simulink model "SWC_HALOUT_type"  (R2021b)
settings: Solver=FixedStepDiscrete  StartTime=0.0  StopTime=10.0  FixedStep=0.005  RelTol=1e-3
undefined symbols (not defined in the file): DIDLen_APPD, DIDLen_APPE, DIDLen_APPPedalZP, DIDLen_APSFunConfig, DIDLen_AutoLock, DIDLen_AutoWipHSpdEN, DIDLen_CALID, DIDLen_CDEODT, DIDLen_CLRDIST, DIDLen_DKCBLESta, DIDLen_DKCKey, DIDLen_DKCSta, DIDLen_DoorNFCAnchorSta, DIDLen_DRLDis, DIDLen_DynoMode, DIDLen_ECUNAME, DIDLen_FDDKCCoordXY, DIDLen_FMHTimer, DIDLen_LFLowPresThre, DIDLen_LFSensorID, DIDLen_LIDAAnchorSta, DIDLen_LRLowPresThre, DIDLen_LRSensorID, DIDLen_MILDIST, DIDLen_NUMPSATRIPSFLTMEMCLR, DIDLen_NVMPedalZP, DIDLen_OBDReq, DIDLen_ODOMETER, DIDLen_PKE, DIDLen_ProtocolId, DIDLen_PSA, DIDLen_QTYPSATRIPS, DIDLen_RFLowPresThre, DIDLen_RFSensorID, DIDLen_RRLowPresThre, DIDLen_RRSensorID, DIDLen_RUNTM, DIDLen_SensorMode, DIDLen_TestGroup, DIDLen_TireSize, DIDLen_TPMSLearnSta, DIDLen_TurnLampFLThreCurr, DIDLen_TurnLampFRThreCurr, DIDLen_TurnLampRLThreCurr, DIDLen_TurnLampRRThreCurr, DIDLen_UIDSta, DIDLen_USSConfig, DIDLen_UWBAnchorSta, DIDLen_VIN, DIDLen_VSS, DIDLen_WhlPres, DIDLen_WhlSensorBattSta, DIDLen_WhlTmp, DIDLen_WipRLSCmdCutFilter, DIDLen_WipRLSCmdHoldFilter, DIDLen_XWDMode, DIDNum_APPD, DIDNum_APPE, DIDNum_APPPedalZP, DIDNum_APSFunConfig ... (+504)
libraries: simulink x893, FVT_lib x320, hdlsllib x6, hcu_lib x5, halout x1
(part 3 of 11)

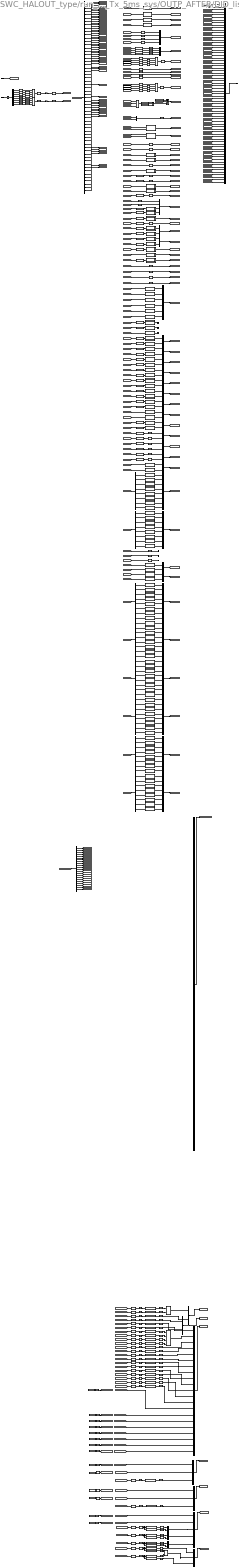
== system SWC_HALOUT_type/run_SWC_HALOUT_Tx_5ms_sys/OUTP_AFTER/DID_list ==
  BOUTP_outputs : Inport
  VHAL_NvmReadArray_raw : Inport  Port=2
  Bit Shift : hdlsllib/Logic and Bit Operations/Bit Shift  mode=Shift Left Logical  N=3
  Bit Shift1 : hdlsllib/Logic and Bit Operations/Bit Shift  mode=Shift Left Logical  N=2
  Bit Shift2 : hdlsllib/Logic and Bit Operations/Bit Shift  mode=Shift Left Logical  N=1
  Bit Shift3 : hdlsllib/Logic and Bit Operations/Bit Shift  mode=Shift Left Logical  N=3
  Bit Shift4 : hdlsllib/Logic and Bit Operations/Bit Shift  mode=Shift Left Logical  N=2
  Bit Shift5 : hdlsllib/Logic and Bit Operations/Bit Shift  mode=Shift Left Logical  N=1
  Bitwise OR : simulink/Logic and Bit Operations/Bitwise Operator  logicop=OR  UseBitMask=off  NumInputPorts=4  BitMask=bin2dec('11011001')  BitMaskRealWorld=Stored Integer
  Bitwise OR1 : simulink/Logic and Bit Operations/Bitwise Operator  logicop=OR  UseBitMask=off  NumInputPorts=4  BitMask=bin2dec('11011001')  BitMaskRealWorld=Stored Integer
  Bitwise OR13 : simulink/Logic and Bit Operations/Bitwise Operator  logicop=OR  UseBitMask=off  NumInputPorts=4  BitMask=bin2dec('00000000000000000000')  BitMaskRealWorld=Stored Integer
  Bitwise OR14 : simulink/Logic and Bit Operations/Bitwise Operator  logicop=OR  UseBitMask=off  NumInputPorts=4  BitMask=bin2dec('00000000000000000000')  BitMaskRealWorld=Stored Integer
  BitwiseAND : simulink/Logic and Bit Operations/Bitwise Operator  logicop=OR  UseBitMask=off  NumInputPorts=2  BitMask=bin2dec('11011001')  BitMaskRealWorld=Stored Integer
  BitwiseAND1 : simulink/Logic and Bit Operations/Bitwise Operator  logicop=OR  UseBitMask=off  NumInputPorts=4  BitMask=bin2dec('11011001')  BitMaskRealWorld=Stored Integer
  BitwiseAND2 : simulink/Logic and Bit Operations/Bitwise Operator  logicop=OR  UseBitMask=off  NumInputPorts=2  BitMask=bin2dec('11011001')  BitMaskRealWorld=Stored Integer
  Bus Creator : BusCreator  Inputs=71
  Bus Selector : BusSelector  OutputSignals=VOUTP_WriteChkLFID_raw,VOUTP_WriteChkRFID_raw,VOUTP_WriteChkLRID_raw,VOUTP_WriteChkRRID_raw,VOUTP_LFWheelPress_raw8,VOUTP_RFWheelPress_raw8,VOUTP_LRWheelPress_raw8,VOUTP_RRWheelPress_raw8,VOUTP_LFWheelTemp_C,VOUTP_RFWheelTemp_C,VOUTP_LRWheelTemp_C,VOUTP_RRWheelTemp_C,VOUTP_LFBatWarn_flg,VOUTP_RFBatWarn_flg,VOUTP_LRBatWarn_flg,VOUTP_RRBatWarn_flg,VOUTP_LFWheelPSW_raw8,VOUTP_LRWheelPSW_raw8,VOUTP_RFWheelPSW_raw8,VOUTP_RRWheelPSW_raw8,VOUTP_LFSensorMode_flg,VOUTP_RFSensorMode_flg,VOUTP_LRSensorMode_flg,VOUTP_RRSensorMode_flg,VOUTP_ALFin_flg,VOUTP_ChkStorge_flg,VOUTP_TPMSStorge_flg,VOUTP_unlearnSfali_flg,VOUTP_WritingCnt_enum,VOUTP_LProgress_enum,VOUTP_EAPS1MIN_pct,VOUTP_EAPS2MIN_pct,VOUTP_DrivetrainSelect_enum,VOUTP_VSS_kph,VOUTP_RUNTM_s,VOUTP_MILDIST_km,VOUTP_CLRDIST_km,VOUTP_APPD_pct,VOUTP_APPE_pct,VOUTP_ODOMETER_km,VOUTP_NUMPSATRIPSFLTMEMCLR_cnt,VOUTP_VinCode_cnt,VOUTP_CALID_cnt,VOUTP_ECUNAME_cnt,VOUTP_PROTOCOLID_enum,VOUTP_PSAR_sec,VOUTP_PSAL_sec,VOUTP_IPSAR_sec,VOUTP_IPSAL_sec,VOUTP_CPSAR_sec,VOUTP_CPSAL_sec,VOUTP_PKER_kphsqr,VOUTP_PKEL_kphsqr,VOUTP_CDEODTR_km,VOUTP_CDEODTL_km,VOUTP_QTYPSATRIPSR_cnt,VOUTP_QTYPSATRIPSL_cnt
  Constant : Constant  Value=ENUM_TPMSLearnStatus_LEARNFAIL
  Constant1 : Constant  Value=ENUM_TPMSLearnStatus_NOTLEARN
  Constant{3..16} (14 alike) : Constant  Value=zeros(10,1)
  Constant2 : Constant  Value=ENUM_TPMSLearnStatus_LEARNED
  Data Type Conversion{,1..58} (59 alike) : DataTypeConversion  OutDataTypeStr=uint8
  Data Type Conversion168 : DataTypeConversion  OutDataTypeStr=single
  Data Type Conversion{169..178} (10 alike) : DataTypeConversion  OutDataTypeStr=uint32
  Data Type Conversion179 : DataTypeConversion  OutDataTypeStr=single
  Demux{,1..8} (9 alike) : Demux  Outputs=8
  Logical Operator1 : Logic  Operator=OR  Inputs=3  AllPortsSameDT=off  OutDataTypeStr=boolean
  Multiply1 : Gain  Gain=1/10000
  Multiply2 : Gain  Gain=1/10000
  Mux : Mux
  Mux{1,4..5,7..19,22..23,37..38,58..60} (23 alike) : Mux  Inputs=2
  Mux2 : Mux
  Mux{20..21,24..29} (8 alike) : Mux  Inputs=8
  Mux3 : Mux
  Mux36 : Mux  Inputs=56
  Mux48 : Mux  Inputs=21
  Mux51 : Mux  Inputs=3
  Mux55 : Mux  Inputs=3
  Mux6 : Mux  Inputs=6
  Mux61 : Mux  Inputs=5
  Mux65 : Mux  Inputs=3
  Selector1 : Selector  InputPortWidth=1024  IndexOptions=Index vector (dialog)  Indices=[112:119]  OutputSizes=1
  Shift Arithmetic37 : ArithShift  BitShiftNumber=8  BitShiftDirection=Left
  Shift Arithmetic38 : ArithShift  BitShiftNumber=16  BitShiftDirection=Left
  Shift Arithmetic39 : ArithShift  BitShiftNumber=24  BitShiftDirection=Left
  Shift Arithmetic40 : ArithShift  BitShiftNumber=8  BitShiftDirection=Left
  Shift Arithmetic41 : ArithShift  BitShiftNumber=16  BitShiftDirection=Left
  Shift Arithmetic42 : ArithShift  BitShiftNumber=24  BitShiftDirection=Left
  SignalPack181 : FVT_lib/hal/SignalPack_shiftAfterMask  RightShiftCnt=0  BitMask=2^4-1  LeftShiftCnt=4
  SignalPack182 : FVT_lib/hal/SignalPack_shiftAfterMask  RightShiftCnt=0  BitMask=2^4-1  LeftShiftCnt=0
  SignalPack{183..186,192..201,302,323} (16 alike) : FVT_lib/hal/SignalPack_shiftAfterMask  RightShiftCnt=0  BitMask=2^8-1  LeftShiftCnt=0
  SignalPack187 : FVT_lib/hal/SignalPack_shiftAfterMask  RightShiftCnt=0  BitMask=2^2-1  LeftShiftCnt=6
  SignalPack188 : FVT_lib/hal/SignalPack_shiftAfterMask  RightShiftCnt=0  BitMask=2^2-1  LeftShiftCnt=4
  SignalPack189 : FVT_lib/hal/SignalPack_shiftAfterMask  RightShiftCnt=0  BitMask=2^2-1  LeftShiftCnt=2
  SignalPack190 : FVT_lib/hal/SignalPack_shiftAfterMask  RightShiftCnt=0  BitMask=2^2-1  LeftShiftCnt=0
  SignalPack191 : FVT_lib/hal/SignalPack_shiftAfterMask  RightShiftCnt=0  BitMask=2^2-1  LeftShiftCnt=0
  SignalPack344 : FVT_lib/hal/SignalPack_shiftAfterMask  RightShiftCnt=8  BitMask=65280  LeftShiftCnt=0
  SignalPack345 : FVT_lib/hal/SignalPack_shiftAfterMask  RightShiftCnt=0  BitMask=255  LeftShiftCnt=0
  SignalPack346 : FVT_lib/hal/SignalPack_shiftAfterMask  RightShiftCnt=8  BitMask=65280  LeftShiftCnt=0
  SignalPack347 : FVT_lib/hal/SignalPack_shiftAfterMask  RightShiftCnt=0  BitMask=255  LeftShiftCnt=0
  SignalPack348 : FVT_lib/hal/SignalPack_shiftAfterMask  RightShiftCnt=8  BitMask=65280  LeftShiftCnt=0
  SignalPack349 : FVT_lib/hal/SignalPack_shiftAfterMask  RightShiftCnt=0  BitMask=255  LeftShiftCnt=0
  SignalPack350 : FVT_lib/hal/SignalPack_shiftAfterMask  RightShiftCnt=1  BitMask=511  LeftShiftCnt=0
  SignalPack351 : FVT_lib/hal/SignalPack_shiftAfterMask  RightShiftCnt=0  BitMask=1  LeftShiftCnt=7
  SignalPack352 : FVT_lib/hal/SignalPack_shiftAfterMask  RightShiftCnt=2  BitMask=508  LeftShiftCnt=0
  SignalPack353 : FVT_lib/hal/SignalPack_shiftAfterMask  RightShiftCnt=0  BitMask=3  LeftShiftCnt=6
  Switch : Switch  Criteria=u2 ~= 0
  Switch1 : Switch  Criteria=u2 ~= 0
  Terminator_{1..6} (6 alike) : Terminator
  UnitConverter{237..278,389..390,413..414,438..439,441..442,444..445,447..448,450..451} (56 alike) : DataTypeConversion  OutDataTypeStr=uint8
  UnitConverter{437,440,443,446,449} (5 alike) : DataTypeConversion  OutDataTypeStr=uint16
  bus_selector : BusSelector  OutputSignals=VOUTP_KeyModeSta_enum,VOUTP_UWBDetArea_enum,VOUTP_BLERSSI_enum,VOUTP_UWBOnOff_flg,VOUTP_UWB1Invalid_flg,VOUTP_UWB2Invalid_flg,VOUTP_UWB3Invalid_flg,VOUTP_UWB4Invalid_flg,VOUTP_UWB0Invalid_flg,VOUTP_UWB1FPP_enum,VOUTP_UWB2FPP_enum,VOUTP_UWB3FPP_enum,VOUTP_UWB4FPP_enum,VOUTP_UWB0FPP_enum,VOUTP_UWB1Distance_enum,VOUTP_UWB2Distance_enum,VOUTP_UWB3Distance_enum,VOUTP_UWB4Distance_enum,VOUTP_UWB0Distance_enum,VOUTP_UIDBatVolt_enum,VOUTP_CoordinateX_enum,VOUTP_CoordinateY_enum
  convert_in{,5..13,17..21,25} (16 alike) : FVT_lib/hal/convert_in  gain=10  offset=0
  convert_in1 : FVT_lib/hal/convert_in  gain=1000  offset=2147483648
  convert_in{14..16,22..24} (6 alike) : FVT_lib/hal/convert_in  gain=1  offset=40
  convert_in2 : FVT_lib/hal/convert_in  gain=1000  offset=2147483648
  convert_in26 : FVT_lib/hal/convert_in  gain=1/0.015625  offset=0
  convert_in{27..30} (4 alike) : FVT_lib/hal/convert_in  gain=2.55  offset=0
  convert_in{3..4,31..32} (4 alike) : FVT_lib/hal/convert_in  gain=1000  offset=0
  convert_in33 : FVT_lib/hal/convert_in  gain=20  offset=0
  convert_in34 : FVT_lib/hal/convert_in  gain=20  offset=0
  convert_in35 : FVT_lib/hal/convert_in  gain=1000000  offset=2147483648
  convert_in36 : FVT_lib/hal/convert_in  gain=1000000  offset=2147483648
  convert_out{,1..3} (4 alike) : FVT_lib/hal/convert_out  gain=1  offset=-40
  convert_out100 : FVT_lib/hal/convert_out  gain=10  offset=-2550
  convert_out101 : FVT_lib/hal/convert_out  gain=10  offset=-2550
  convert_out{56..59,61..67,90,94} (13 alike) : FVT_lib/hal/convert_out  gain=1  offset=0
  convert_out{68..70,72..73} (5 alike) : FVT_lib/hal/convert_out  gain=1  offset=-127
  convert_out{74..78,97..99} (8 alike) : FVT_lib/hal/convert_out  gain=10  offset=0
  pct2raw1 : Subsystem
  pct2raw8 : Subsystem
  uint16Touint8Array1 : Subsystem
  uint16Touint8Array10 : Subsystem
  uint16Touint8Array11 : Subsystem
  uint16Touint8Array12 : Subsystem
  uint16Touint8Array13 : Subsystem
  uint16Touint8Array14 : Subsystem
  uint16Touint8Array15 : Subsystem
  uint16Touint8Array16 : Subsystem
  uint16Touint8Array17 : Subsystem
  uint16Touint8Array18 : Subsystem
  uint16Touint8Array19 : Subsystem
  uint16Touint8Array2 : Subsystem
  uint16Touint8Array20 : Subsystem
  uint16Touint8Array21 : Subsystem
  uint16Touint8Array22 : Subsystem
  uint16Touint8Array23 : Subsystem
  uint16Touint8Array24 : Subsystem
  uint16Touint8Array25 : Subsystem
  uint16Touint8Array26 : Subsystem
  uint16Touint8Array27 : Subsystem
  uint16Touint8Array28 : Subsystem
  uint16Touint8Array29 : Subsystem
  uint16Touint8Array3 : Subsystem
  uint16Touint8Array4 : Subsystem
  uint16Touint8Array5 : Subsystem
  uint16Touint8Array6 : Subsystem
  uint16Touint8Array7 : Subsystem
  uint16Touint8Array8 : Subsystem
  uint16Touint8Array9 : Subsystem
  uint32Touint8Array : Subsystem
  uint32Touint8Array1 : Subsystem
  uint32Touint8Array10 : Subsystem
  uint32Touint8Array11 : Subsystem
  uint32Touint8Array12 : Subsystem
  uint32Touint8Array13 : Subsystem
  uint32Touint8Array14 : Subsystem
  uint32Touint8Array15 : Subsystem
  uint32Touint8Array16 : Subsystem
  uint32Touint8Array17 : Subsystem
  uint32Touint8Array18 : Subsystem
  uint32Touint8Array19 : Subsystem
  uint32Touint8Array2 : Subsystem
  uint32Touint8Array20 : Subsystem
  uint32Touint8Array21 : Subsystem
  uint32Touint8Array22 : Subsystem
  uint32Touint8Array23 : Subsystem
  uint32Touint8Array24 : Subsystem
  uint32Touint8Array25 : Subsystem
  uint32Touint8Array26 : Subsystem
  uint32Touint8Array27 : Subsystem
  uint32Touint8Array28 : Subsystem
  uint32Touint8Array29 : Subsystem
  uint32Touint8Array3 : Subsystem
  uint32Touint8Array30 : Subsystem
  uint32Touint8Array31 : Subsystem
  uint32Touint8Array32 : Subsystem
  uint32Touint8Array33 : Subsystem
  uint32Touint8Array34 : Subsystem
  uint32Touint8Array35 : Subsystem
  uint32Touint8Array36 : Subsystem
  uint32Touint8Array37 : Subsystem
  uint32Touint8Array38 : Subsystem
  uint32Touint8Array39 : Subsystem
  uint32Touint8Array4 : Subsystem
  uint32Touint8Array40 : Subsystem
  uint32Touint8Array41 : Subsystem
  uint32Touint8Array42 : Subsystem
  uint32Touint8Array43 : Subsystem
  uint32Touint8Array44 : Subsystem
  uint32Touint8Array45 : Subsystem
  uint32Touint8Array46 : Subsystem
  uint32Touint8Array47 : Subsystem
  uint32Touint8Array48 : Subsystem
  uint32Touint8Array49 : Subsystem
  uint32Touint8Array5 : Subsystem
  uint32Touint8Array50 : Subsystem
  uint32Touint8Array51 : Subsystem
  uint32Touint8Array52 : Subsystem
  uint32Touint8Array53 : Subsystem
  uint32Touint8Array54 : Subsystem
  uint32Touint8Array55 : Subsystem
  uint32Touint8Array56 : Subsystem
  uint32Touint8Array57 : Subsystem
  uint32Touint8Array58 : Subsystem
  uint32Touint8Array59 : Subsystem
  uint32Touint8Array6 : Subsystem
  uint32Touint8Array60 : Subsystem
  uint32Touint8Array61 : Subsystem
  uint32Touint8Array62 : Subsystem
  uint32Touint8Array63 : Subsystem
  uint32Touint8Array64 : Subsystem
  uint32Touint8Array65 : Subsystem
  uint32Touint8Array66 : Subsystem
  uint32Touint8Array67 : Subsystem
  uint32Touint8Array68 : Subsystem
  uint32Touint8Array69 : Subsystem
  uint32Touint8Array7 : Subsystem
  uint32Touint8Array70 : Subsystem
  uint32Touint8Array71 : Subsystem
  uint32Touint8Array72 : Subsystem
  uint32Touint8Array73 : Subsystem
  uint32Touint8Array74 : Subsystem
  uint32Touint8Array75 : Subsystem
  uint32Touint8Array76 : Subsystem
  uint32Touint8Array77 : Subsystem
  uint32Touint8Array78 : Subsystem
  uint32Touint8Array79 : Subsystem
  uint32Touint8Array8 : Subsystem
  uint32Touint8Array80 : Subsystem
  uint32Touint8Array81 : Subsystem
  uint32Touint8Array82 : Subsystem
  uint32Touint8Array83 : Subsystem
  uint32Touint8Array84 : Subsystem
  uint32Touint8Array85 : Subsystem
  uint32Touint8Array86 : Subsystem
  uint32Touint8Array9 : Subsystem
  BOUTP_DIDSetData_outputs : Outport
  wires:
  Bus Selector/1 -> [VOUTP_WriteChkLFID_raw]  "<VOUTP_WriteChkLFID_raw>"
  Bus Selector/2 -> [VOUTP_WriteChkRFID_raw]  "<VOUTP_WriteChkRFID_raw>"
  Bus Selector/4 -> [VOUTP_WriteChkRRID_raw]  "<VOUTP_WriteChkRRID_raw>"
  Bus Selector/3 -> [VOUTP_WriteChkLRID_raw]  "<VOUTP_WriteChkLRID_raw>"
  Bus Selector/5 -> [VOUTP_LFWheelPress_raw8]  "<VOUTP_LFWheelPress_raw8>"
  Bus Selector/6 -> [VOUTP_RFWheelPress_raw8]  "<VOUTP_RFWheelPress_raw8>"
  Bus Selector/7 -> [VOUTP_LRWheelPress_raw8]  "<VOUTP_LRWheelPress_raw8>"
  Bus Selector/8 -> [VOUTP_RRWheelPress_raw8]  "<VOUTP_RRWheelPress_raw8>"
  Bus Selector/13 -> [VOUTP_LFBatWarn_flg]  "<VOUTP_LFBatWarn_flg>"
  Bus Selector/14 -> [VOUTP_RFBatWarn_flg]  "<VOUTP_RFBatWarn_flg>"
  Bus Selector/15 -> [VOUTP_LRBatWarn_flg]  "<VOUTP_LRBatWarn_flg>"
  Bus Selector/16 -> [VOUTP_RRBatWarn_flg]  "<VOUTP_RRBatWarn_flg>"
  Bus Selector/18 -> [VOUTP_LRWheelPSW_raw8]  "<VOUTP_LRWheelPSW_raw8>"
  Bus Selector/19 -> [VOUTP_RFWheelPSW_raw8]  "<VOUTP_RFWheelPSW_raw8>"
  Bus Selector/20 -> [VOUTP_RRWheelPSW_raw8]  "<VOUTP_RRWheelPSW_raw8>"
  Bus Selector/17 -> [VOUTP_LFWheelPSW_raw8]  "<VOUTP_LFWheelPSW_raw8>"
  Bus Selector/21 -> [VOUTP_LFSensorMode_flg]  "<VOUTP_LFSensorMode_flg>"
  Bus Selector/22 -> [VOUTP_RFSensorMode_flg]  "<VOUTP_RFSensorMode_flg>"
  Bus Selector/23 -> [VOUTP_LRSensorMode_flg]  "<VOUTP_LRSensorMode_flg>"
  Bus Selector/24 -> [VOUTP_RRSensorMode_flg]  "<VOUTP_RRSensorMode_flg>"
  Bus Selector/27 -> [VOUTP_TPMSStorge_flg]  "<VOUTP_TPMSStorge_flg>"
  Bus Selector/25 -> [VOUTP_ALFin_flg]  "<VOUTP_ALFin_flg>"
  Bus Selector/26 -> [VOUTP_ChkStorge_flg]  "<VOUTP_ChkStorge_flg>"
  Bus Selector/28 -> [VOUTP_unlearnSfali_flg]  "<VOUTP_unlearnSfali_flg>"
  Bus Selector/9 -> [VOUTP_LFWheelTemp_C]  "<VOUTP_LFWheelTemp_C>"
  Bus Selector/10 -> [VOUTP_RFWheelTemp_C]  "<VOUTP_RFWheelTemp_C>"
  Bus Selector/11 -> [VOUTP_LRWheelTemp_C]  "<VOUTP_LRWheelTemp_C>"
  Bus Selector/12 -> [VOUTP_RRWheelTemp_C]  "<VOUTP_RRWheelTemp_C>"
  Data Type Conversion8/1 -> Mux2/1
  Data Type Conversion9/1 -> Mux2/2
  Data Type Conversion10/1 -> Mux2/3
  Data Type Conversion11/1 -> Mux2/4
  [VOUTP_LFWheelPSW_raw8] -> Data Type Conversion6/1
  [VOUTP_RRWheelPSW_raw8] -> Data Type Conversion5/1
  [VOUTP_LFSensorMode_flg] -> Data Type Conversion21/1
  [VOUTP_RRSensorMode_flg] -> Data Type Conversion14/1
  [VOUTP_LRSensorMode_flg] -> Data Type Conversion12/1
  [VOUTP_RFSensorMode_flg] -> Data Type Conversion13/1
  Data Type Conversion21/1 -> Bitwise OR/1
  Data Type Conversion12/1 -> Bit Shift1/1
  Data Type Conversion14/1 -> Bit Shift/1
  Constant1/1 -> Switch1/3
  [VOUTP_ALFin_flg] -> Logical Operator1/1
  Switch1/1 -> Switch/3
  [VOUTP_ChkStorge_flg] -> Logical Operator1/2
  Constant/1 -> Switch/1
  Constant2/1 -> Switch1/1
  [VOUTP_TPMSStorge_flg] -> Logical Operator1/3
  Logical Operator1/1 -> Switch1/2
  [VOUTP_unlearnSfali_flg] -> Switch/2
  Mux/1 -> [VHAL_DIDSetWhlPres_raw8]
  Mux2/1 -> [VHAL_DIDSetWhlTmp_raw8]
  Data Type Conversion6/1 -> [VHAL_DIDSetLFLowPresThre_raw8]
  Data Type Conversion7/1 -> [VHAL_DIDSetRFLowPresThre_raw8]
  Data Type Conversion4/1 -> [VHAL_DIDSetLRLowPresThre_raw8]
  Data Type Conversion5/1 -> [VHAL_DIDSetRRLowPresThre_raw8]
  Bitwise OR/1 -> Data Type Conversion20/1
  Switch/1 -> [VHAL_DIDSetTPMSLearnSta_raw8]
  Bit Shift/1 -> Bitwise OR/4
  Bit Shift1/1 -> Bitwise OR/3
  Bit Shift2/1 -> Bitwise OR/2
  Data Type Conversion20/1 -> [VHAL_DIDSetSensorMode_raw8]
  Data Type Conversion13/1 -> Bit Shift2/1
  [VOUTP_RFBatWarn_flg] -> Data Type Conversion2/1
  Data Type Conversion1/1 -> Bit Shift4/1
  [VOUTP_LRBatWarn_flg] -> Data Type Conversion1/1
  [VOUTP_LFBatWarn_flg] -> Data Type Conversion22/1
  Bitwise OR1/1 -> Data Type Conversion15/1
  Bit Shift4/1 -> Bitwise OR1/3
  Data Type Conversion2/1 -> Bit Shift5/1
  Bit Shift3/1 -> Bitwise OR1/4
  Data Type Conversion22/1 -> Bitwise OR1/1
  Data Type Conversion3/1 -> Bit Shift3/1
  Bit Shift5/1 -> Bitwise OR1/2
  [VOUTP_RRBatWarn_flg] -> Data Type Conversion3/1
  Data Type Conversion15/1 -> [VHAL_DIDSetWhlSensorBattSta_raw8]
  [VHAL_DIDSetTPMSLearnSta_raw8] -> Bus Creator/13  "VHAL_DIDSetTPMSLearnSta_raw8"
  [VHAL_DIDSetLFSensorID_raw8] -> Bus Creator/1  "VHAL_DIDSetLFSensorID_raw8"
  [VHAL_DIDSetRFSensorID_raw8] -> Bus Creator/2  "VHAL_DIDSetRFSensorID_raw8"
  [VHAL_DIDSetLRSensorID_raw8] -> Bus Creator/3  "VHAL_DIDSetLRSensorID_raw8"
  [VHAL_DIDSetRRSensorID_raw8] -> Bus Creator/4  "VHAL_DIDSetRRSensorID_raw8"
  [VHAL_DIDSetWhlPres_raw8] -> Bus Creator/5  "VHAL_DIDSetWhlPres_raw8"
  [VHAL_DIDSetWhlTmp_raw8] -> Bus Creator/6  "VHAL_DIDSetWhlTmp_raw8"
  [VHAL_DIDSetWhlSensorBattSta_raw8] -> Bus Creator/7  "VHAL_DIDSetWhlSensorBattSta_raw8"
  [VHAL_DIDSetLFLowPresThre_raw8] -> Bus Creator/8  "VHAL_DIDSetLFLowPresThre_raw8"
  [VHAL_DIDSetRFLowPresThre_raw8] -> Bus Creator/9  "VHAL_DIDSetRFLowPresThre_raw8"
  [VHAL_DIDSetLRLowPresThre_raw8] -> Bus Creator/10  "VHAL_DIDSetLRLowPresThre_raw8"
  [VHAL_DIDSetRRLowPresThre_raw8] -> Bus Creator/11  "VHAL_DIDSetRRLowPresThre_raw8"
  [VHAL_DIDSetSensorMode_raw8] -> Bus Creator/12  "VHAL_DIDSetSensorMode_raw8"
  Bus Creator/1 -> BOUTP_DIDSetData_outputs/1
  [VOUTP_WriteChkLFID_raw] -> uint32Touint8Array/1(In1)
  uint32Touint8Array/1(Out1) -> [VHAL_DIDSetLFSensorID_raw8]
  [VOUTP_WriteChkRFID_raw] -> uint32Touint8Array1/1(In1)
  uint32Touint8Array1/1(Out1) -> [VHAL_DIDSetRFSensorID_raw8]
  [VOUTP_WriteChkLRID_raw] -> uint32Touint8Array2/1(In1)
  uint32Touint8Array2/1(Out1) -> [VHAL_DIDSetLRSensorID_raw8]
  [VOUTP_WriteChkRRID_raw] -> uint32Touint8Array3/1(In1)
  uint32Touint8Array3/1(Out1) -> [VHAL_DIDSetRRSensorID_raw8]
  [VOUTP_RFWheelPress_raw8] -> Data Type Conversion17/1
  [VOUTP_LFWheelPress_raw8] -> Data Type Conversion16/1
  [VOUTP_LRWheelPress_raw8] -> Data Type Conversion18/1
  [VOUTP_RRWheelPress_raw8] -> Data Type Conversion19/1
  convert_out/1 -> Data Type Conversion8/1
  convert_out1/1 -> Data Type Conversion9/1
  convert_out2/1 -> Data Type Conversion10/1
  convert_out3/1 -> Data Type Conversion11/1
  Data Type Conversion16/1 -> Mux/1
  Data Type Conversion17/1 -> Mux/2
  Data Type Conversion18/1 -> Mux/3
  Data Type Conversion19/1 -> Mux/4
  [VOUTP_LFWheelTemp_C] -> convert_out/1
  [VOUTP_RFWheelTemp_C] -> convert_out1/1
  [VOUTP_LRWheelTemp_C] -> convert_out2/1
  [VOUTP_RRWheelTemp_C] -> convert_out3/1
  [VOUTP_RFWheelPSW_raw8] -> Data Type Conversion7/1
  [VOUTP_LRWheelPSW_raw8] -> Data Type Conversion4/1
  Bus Selector/29 -> [VOUTP_WritingCnt_enum]  "<VOUTP_WritingCnt_enum>"
  Bus Selector/30 -> [VOUTP_LProgress_enum]  "<VOUTP_LProgress_enum>"
  [VOUTP_WritingCnt_enum] -> Mux1/2
  [VHAL_TPMSSensorIDRegResults_raw8] -> Bus Creator/14  "VHAL_TPMSSensorIDRegResults_raw8"
  Data Type Conversion23/1 -> [VHAL_TPMSSensorIDRegResults_raw8]
  [VOUTP_LProgress_enum] -> Mux1/1
  Mux1/1 -> Data Type Conversion23/1
  pct2raw8/1(PedalZP_raw8) -> [VHAL_DIDSetAPPPedalZP_raw8]
  pct2raw1/1(PedalZP_raw8) -> [VHAL_DIDSetNVMPedalZP_raw8]
  [VHAL_DIDSetAPPPedalZP_raw8] -> Bus Creator/15  "VHAL_DIDSetAPPPedalZP_raw8"
  [VHAL_DIDSetNVMPedalZP_raw8] -> Bus Creator/16  "VHAL_DIDSetNVMPedalZP_raw8"
  Data Type Conversion174/1 -> Bitwise OR14/1
  Demux/7 -> Data Type Conversion176/1
  Data Type Conversion170/1 -> Shift Arithmetic37/1
  Demux/2 -> Data Type Conversion170/1
  Data Type Conversion168/1 -> [VHAL_EAPS2MINMem_pct]
  Data Type Conversion172/1 -> Shift Arithmetic39/1
  Data Type Conversion169/1 -> Bitwise OR13/1
  Data Type Conversion175/1 -> Shift Arithmetic40/1
  Data Type Conversion176/1 -> Shift Arithmetic41/1
  Data Type Conversion173/1 -> Multiply1/1
  Data Type Conversion177/1 -> Shift Arithmetic42/1
  Data Type Conversion178/1 -> Multiply2/1
  Multiply2/1 -> Data Type Conversion168/1
  Data Type Conversion171/1 -> Shift Arithmetic38/1
  Demux/8 -> Data Type Conversion177/1
  Demux/5 -> Data Type Conversion174/1
  Demux/6 -> Data Type Conversion175/1
  Bitwise OR13/1 -> Data Type Conversion173/1
  Shift Arithmetic41/1 -> Bitwise OR14/3
  Demux/3 -> Data Type Conversion171/1
  Bitwise OR14/1 -> Data Type Conversion178/1
  Shift Arithmetic39/1 -> Bitwise OR13/4
  Multiply1/1 -> Data Type Conversion179/1
  Shift Arithmetic38/1 -> Bitwise OR13/3
  Demux/4 -> Data Type Conversion172/1
  Data Type Conversion179/1 -> [VHAL_EAPS1MINMem_pct]
  Shift Arithmetic42/1 -> Bitwise OR14/4
  Shift Arithmetic40/1 -> Bitwise OR14/2
  Shift Arithmetic37/1 -> Bitwise OR13/2
  Demux/1 -> Data Type Conversion169/1
  Selector1/1 -> Demux/1
  VHAL_NvmReadArray_raw/1 -> Selector1/1
  Bus Selector/31 -> [VOUTP_EAPS1MIN_pct]  "<VOUTP_EAPS1MIN_pct>"
  Bus Selector/32 -> [VOUTP_EAPS2MIN_pct]  "<VOUTP_EAPS2MIN_pct>"
  [VOUTP_EAPS1MIN_pct] -> pct2raw8/1(EAPS1_pct)
  [VOUTP_EAPS2MIN_pct] -> pct2raw8/2(EAPS2_pct)
  [VHAL_EAPS1MINMem_pct] -> pct2raw1/1(EAPS1_pct)
  [VHAL_EAPS2MINMem_pct] -> pct2raw1/2(EAPS2_pct)
  Bus Selector/33 -> [VOUTP_DrivetrainSelect_enum]  "<VOUTP_DrivetrainSelect_enum>"
  [VOUTP_DrivetrainSelect_enum] -> Data Type Conversion24/1
  Data Type Conversion24/1 -> [VHAL_DIDSetXWDMode_raw8]
  [VHAL_DIDSetXWDMode_raw8] -> Bus Creator/17  "VHAL_DIDSetXWDMode_raw8"
  Bus Selector/41 -> [VOUTP_NUMPSATRIPSFLTMEMCLR_cnt]  "<VOUTP_NUMPSATRIPSFLTMEMCLR_cnt>"
  Bus Selector/42 -> [VOUTP_VinCode_cnt]  "<VOUTP_VinCode_cnt>"
  Bus Selector/43 -> [VOUTP_CALID_cnt]  "<VOUTP_CALID_cnt>"
  Bus Selector/44 -> [VOUTP_ECUNAME_cnt]  "<VOUTP_ECUNAME_cnt>"
  Bus Selector/45 -> [VOUTP_PROTOCOLID_enum]  "<VOUTP_PROTOCOLID_enum>"
  Bus Selector/46 -> [VOUTP_PSAR_sec]  "<VOUTP_PSAR_sec>"
  Bus Selector/47 -> [VOUTP_PSAL_sec]  "<VOUTP_PSAL_sec>"
  Bus Selector/48 -> [VOUTP_IPSAR_sec]  "<VOUTP_IPSAR_sec>"
  Bus Selector/49 -> [VOUTP_IPSAL_sec]  "<VOUTP_IPSAL_sec>"
  Bus Selector/50 -> [VOUTP_CPSAR_sec]  "<VOUTP_CPSAR_sec>"
  Bus Selector/51 -> [VOUTP_CPSAL_sec]  "<VOUTP_CPSAL_sec>"
  Bus Selector/34 -> [VOUTP_VSS_kph]  "<VOUTP_VSS_kph>"
  Bus Selector/35 -> [VOUTP_RUNTM_s]  "<VOUTP_RUNTM_s>"
  Bus Selector/36 -> [VOUTP_MILDIST_km]  "<VOUTP_MILDIST_km>"
  Bus Selector/37 -> [VOUTP_CLRDIST_km]  "<VOUTP_CLRDIST_km>"
  Bus Selector/38 -> [VOUTP_APPD_pct]  "<VOUTP_APPD_pct>"
  Bus Selector/39 -> [VOUTP_APPE_pct]  "<VOUTP_APPE_pct>"
  Bus Selector/40 -> [VOUTP_ODOMETER_km]  "<VOUTP_ODOMETER_km>"
  Bus Selector/57 -> [VOUTP_QTYPSATRIPSL_cnt]  "<VOUTP_QTYPSATRIPSL_cnt>"
  Bus Selector/52 -> [VOUTP_PKER_kphsqr]  "<VOUTP_PKER_kphsqr>"
  Bus Selector/53 -> [VOUTP_PKEL_kphsqr]  "<VOUTP_PKEL_kphsqr>"
  Bus Selector/54 -> [VOUTP_CDEODTR_km]  "<VOUTP_CDEODTR_km>"
  Bus Selector/55 -> [VOUTP_CDEODTL_km]  "<VOUTP_CDEODTL_km>"
  Bus Selector/56 -> [VOUTP_QTYPSATRIPSR_cnt]  "<VOUTP_QTYPSATRIPSR_cnt>"
  [VOUTP_VSS_kph] -> Data Type Conversion25/1
  Data Type Conversion25/1 -> [VHAL_DIDSetVSS_raw8]
  [VOUTP_RUNTM_s] -> uint16Touint8Array2/1(In1)
  [VOUTP_MILDIST_km] -> uint16Touint8Array1/1(In1)
  [VOUTP_WARMUPS_cnt] -> Data Type Conversion26/1
  [VOUTP_CLRDIST_km] -> uint16Touint8Array3/1(In1)
  [VOUTP_MILTIME_min] -> uint16Touint8Array4/1(In1)
  [VOUTP_CLRTIME_min] -> uint16Touint8Array5/1(In1)
  [VOUTP_STASUP_enum] -> Data Type Conversion30/1
  [VOUTP_HEVMODE_enum] -> Data Type Conversion31/1
  uint16Touint8Array6/1(Out1) -> Mux3/3
  uint16Touint8Array7/1(Out1) -> Mux3/4
  Data Type Conversion30/1 -> Mux3/1
  Data Type Conversion31/1 -> Mux3/2
  [VOUTP_NUMPSATRIPSFLTMEMCLR_cnt] -> uint16Touint8Array12/1(In1)
  [VOUTP_VinCode_cnt] -> Data Type Conversion33/1
  [VOUTP_CALID_cnt] -> Data Type Conversion34/1
  [VOUTP_ECUNAME_cnt] -> Data Type Conversion35/1
  [VOUTP_PROTOCOLID_enum] -> Data Type Conversion36/1
  [VOUTP_PSAR_sec] -> uint32Touint8Array7/1(In1)
  [VOUTP_PSAL_sec] -> uint32Touint8Array8/1(In1)
  [VOUTP_IPSAR_sec] -> uint32Touint8Array9/1(In1)
  [VOUTP_IPSAL_sec] -> uint32Touint8Array10/1(In1)
  [VOUTP_CPSAR_sec] -> uint32Touint8Array12/1(In1)
  [VOUTP_CPSAL_sec] -> uint32Touint8Array11/1(In1)
  [VOUTP_IGNCNTR_cnt] -> uint16Touint8Array13/1(In1)
  convert_in3/1 -> uint32Touint8Array15/1(In1)
  convert_in4/1 -> uint32Touint8Array16/1(In1)
  convert_in19/1 -> uint32Touint8Array17/1(In1)
  convert_in18/1 -> uint32Touint8Array18/1(In1)
  convert_in17/1 -> uint32Touint8Array20/1(In1)
  convert_in5/1 -> uint32Touint8Array19/1(In1)
  convert_in6/1 -> uint32Touint8Array21/1(In1)
  convert_in7/1 -> uint32Touint8Array22/1(In1)
  convert_in8/1 -> uint32Touint8Array23/1(In1)
  convert_in9/1 -> uint32Touint8Array24/1(In1)
  convert_in20/1 -> uint32Touint8Array25/1(In1)
  convert_in21/1 -> uint32Touint8Array26/1(In1)
  convert_in10/1 -> uint32Touint8Array27/1(In1)
  convert_in11/1 -> uint32Touint8Array28/1(In1)
  [VOUTP_PKER_kphsqr] -> uint32Touint8Array29/1(In1)
  [VOUTP_PKEL_kphsqr] -> uint32Touint8Array30/1(In1)
  convert_in12/1 -> uint32Touint8Array31/1(In1)
  convert_in13/1 -> uint32Touint8Array32/1(In1)
  [VOUTP_QTYPSATRIPSR_cnt] -> uint32Touint8Array33/1(In1)
  [VOUTP_QTYPSATRIPSL_cnt] -> uint32Touint8Array34/1(In1)
  [VOUTP_RESSCNTDODRNGR_cnt] -> Demux1/1
  Demux1/1 -> uint16Touint8Array14/1(In1)
  Demux1/2 -> uint16Touint8Array15/1(In1)
  Demux1/3 -> uint16Touint8Array16/1(In1)
  Demux1/4 -> uint16Touint8Array17/1(In1)
  Demux1/5 -> uint16Touint8Array18/1(In1)
  Demux1/6 -> uint16Touint8Array19/1(In1)
  Demux1/7 -> uint16Touint8Array20/1(In1)
  Demux1/8 -> uint16Touint8Array21/1(In1)
  Demux2/8 -> uint16Touint8Array29/1(In1)
  Demux2/7 -> uint16Touint8Array28/1(In1)
  Demux2/6 -> uint16Touint8Array27/1(In1)
  Demux2/5 -> uint16Touint8Array26/1(In1)
  Demux2/4 -> uint16Touint8Array25/1(In1)
  Demux2/3 -> uint16Touint8Array24/1(In1)
  Demux2/2 -> uint16Touint8Array23/1(In1)
  Demux2/1 -> uint16Touint8Array22/1(In1)
  [VOUTP_RESSCNTDODRNGL_cnt] -> Demux2/1
  [VOUTP_RESSTTEMPRNGAXIS_enum] -> Data Type Conversion43/1
  [VOUTP_RESSTIMESOCRNGAXIS_enum] -> Data Type Conversion44/1
  [VOUTP_RESSCNTSDODRNGAXIS_enum] -> Data Type Conversion45/1
  [VOUTP_ETMATOER_kWh] -> uint32Touint8Array35/1(In1)
  [VOUTP_ETMATOEL_kWh] -> uint32Touint8Array36/1(In1)
  [VOUTP_ETMBTOER_kWh] -> uint32Touint8Array37/1(In1)
  [VOUTP_ETMBTOEL_kWh] -> uint32Touint8Array38/1(In1)
  [VOUTP_RESSTIMESOCPSARNGR_s] -> Demux3/1
  Demux3/1 -> uint32Touint8Array39/1(In1)
  Demux3/2 -> uint32Touint8Array40/1(In1)
  Demux3/3 -> uint32Touint8Array41/1(In1)
  Demux3/4 -> uint32Touint8Array42/1(In1)
  Demux3/5 -> uint32Touint8Array43/1(In1)
  Demux3/6 -> uint32Touint8Array44/1(In1)
  Demux3/7 -> uint32Touint8Array45/1(In1)
  Demux3/8 -> uint32Touint8Array46/1(In1)
  Demux4/8 -> uint32Touint8Array54/1(In1)
  Demux4/7 -> uint32Touint8Array53/1(In1)
  Demux4/6 -> uint32Touint8Array52/1(In1)
  Demux4/5 -> uint32Touint8Array51/1(In1)
  Demux4/4 -> uint32Touint8Array50/1(In1)
  Demux4/3 -> uint32Touint8Array49/1(In1)
  Demux4/2 -> uint32Touint8Array48/1(In1)
  Demux4/1 -> uint32Touint8Array47/1(In1)
  [VOUTP_RESSTIMESOCPSARNGL_s] -> Demux4/1
  [VOUTP_RESSTIMESOCCHGRNGL_s] -> Demux6/1
  Demux6/1 -> uint32Touint8Array63/1(In1)
  Demux6/2 -> uint32Touint8Array64/1(In1)
  Demux6/3 -> uint32Touint8Array65/1(In1)
  Demux6/4 -> uint32Touint8Array66/1(In1)
  Demux6/5 -> uint32Touint8Array67/1(In1)
  Demux6/6 -> uint32Touint8Array68/1(In1)
  Demux6/7 -> uint32Touint8Array69/1(In1)
  Demux6/8 -> uint32Touint8Array70/1(In1)
  Demux5/8 -> uint32Touint8Array62/1(In1)
  Demux5/7 -> uint32Touint8Array61/1(In1)
  Demux5/6 -> uint32Touint8Array60/1(In1)
  Demux5/5 -> uint32Touint8Array59/1(In1)
  Demux5/4 -> uint32Touint8Array58/1(In1)
  Demux5/3 -> uint32Touint8Array57/1(In1)
  Demux5/2 -> uint32Touint8Array56/1(In1)
  Demux5/1 -> uint32Touint8Array55/1(In1)
  [VOUTP_RESSTIMESOCCHGRNGR_s] -> Demux5/1
  [VOUTP_RESSTIMESOCOFFRNGR_s] -> Demux7/1
  Demux7/1 -> uint32Touint8Array71/1(In1)
  Demux7/2 -> uint32Touint8Array72/1(In1)
  Demux7/3 -> uint32Touint8Array73/1(In1)
  Demux7/4 -> uint32Touint8Array74/1(In1)
  Demux7/5 -> uint32Touint8Array75/1(In1)
  Demux7/6 -> uint32Touint8Array76/1(In1)
  Demux7/7 -> uint32Touint8Array77/1(In1)
  Demux7/8 -> uint32Touint8Array78/1(In1)
  Demux8/8 -> uint32Touint8Array86/1(In1)
  Demux8/7 -> uint32Touint8Array85/1(In1)
  Demux8/6 -> uint32Touint8Array84/1(In1)
  Demux8/5 -> uint32Touint8Array83/1(In1)
  Demux8/4 -> uint32Touint8Array82/1(In1)
  Demux8/3 -> uint32Touint8Array81/1(In1)
  Demux8/2 -> uint32Touint8Array80/1(In1)
  Demux8/1 -> uint32Touint8Array79/1(In1)
  [VOUTP_RESSTIMESOCOFFRNGL_s] -> Demux8/1
  uint16Touint8Array2/1(Out1) -> [VHAL_DIDSetRUNTM_raw8]
  uint16Touint8Array1/1(Out1) -> [VHAL_DIDSetMILDIST_raw8]
  Data Type Conversion26/1 -> [VHAL_DIDSetWARMUPS_raw8]
  uint16Touint8Array3/1(Out1) -> [VHAL_DIDSetCLRDIST_raw8]
  Data Type Conversion27/1 -> [VHAL_DIDSetAPPD_raw8]
  Data Type Conversion29/1 -> [VHAL_DIDSetAPPE_raw8]
  uint16Touint8Array4/1(Out1) -> [VHAL_DIDSetMILTIME_raw8]
  uint16Touint8Array5/1(Out1) -> [VHAL_DIDSetCLRTIME_raw8]
  Data Type Conversion28/1 -> [VHAL_DIDSetBATSOC_raw8]
  Mux3/1 -> [VHAL_DIDSetHEVVehSysData_raw8]
  uint32Touint8Array4/1(Out1) -> [VHAL_DIDSetODOMETER_raw8]
  Data Type Conversion32/1 -> [VHAL_DIDSetBATSOH_raw8]
  uint16Touint8Array9/1(Out1) -> Mux4/2
  uint16Touint8Array8/1(Out1) -> Mux4/1
  Mux4/1 -> [VHAL_DIDSetHVBCellVoltMinMax_raw8]
  uint16Touint8Array10/1(Out1) -> Mux5/1
  uint16Touint8Array11/1(Out1) -> Mux5/2
  Mux5/1 -> [VHAL_DIDSetHVESSCHARGE_raw8]
  uint32Touint8Array5/1(Out1) -> [VHAL_DIDSetHVESSENER_raw8]
  uint16Touint8Array12/1(Out1) -> [VHAL_DIDSetNUMPSATRIPSFLTMEMCLR_raw8]
  uint32Touint8Array6/1(Out1) -> [VHAL_DIDSetHVBattCurr_raw8]
  Data Type Conversion33/1 -> [VHAL_DIDSetVIN_raw8]
  Data Type Conversion34/1 -> [VHAL_DIDSetCALID_raw8]
  Data Type Conversion35/1 -> [VHAL_DIDSetECUNAME_raw8]
  Data Type Conversion36/1 -> [VHAL_DIDSetProtocolId_raw8]
  uint32Touint8Array7/1(Out1) -> Mux6/1
  uint32Touint8Array8/1(Out1) -> Mux6/2
  uint32Touint8Array9/1(Out1) -> Mux6/3
  uint32Touint8Array10/1(Out1) -> Mux6/4
  uint32Touint8Array12/1(Out1) -> Mux6/5
  uint32Touint8Array11/1(Out1) -> Mux6/6
  Mux6/1 -> [VHAL_DIDSetPSA_raw8]
  uint32Touint8Array15/1(Out1) -> Mux7/1
  uint32Touint8Array16/1(Out1) -> Mux7/2
  Mux7/1 -> [VHAL_DIDSetTNBCPSA_raw8]
  Mux8/1 -> [VHAL_DIDSetTNECPSA_raw8]
  uint32Touint8Array18/1(Out1) -> Mux8/2
  uint32Touint8Array17/1(Out1) -> Mux8/1
  uint32Touint8Array21/1(Out1) -> Mux10/1
  uint32Touint8Array22/1(Out1) -> Mux10/2
  Mux10/1 -> [VHAL_DIDSetTGEOVC_raw8]
  Mux9/1 -> [VHAL_DIDSetTEBPSA_raw8]
  uint32Touint8Array20/1(Out1) -> Mux9/2
  uint32Touint8Array19/1(Out1) -> Mux9/1
  uint32Touint8Array23/1(Out1) -> Mux12/1
  uint32Touint8Array24/1(Out1) -> Mux12/2
  Mux12/1 -> [VHAL_DIDSetGECHGOVCDC_raw8]
  Mux11/1 -> [VHAL_DIDSetGECHGOVCAC_raw8]
  uint32Touint8Array26/1(Out1) -> Mux11/2
  uint32Touint8Array25/1(Out1) -> Mux11/1
  uint32Touint8Array27/1(Out1) -> Mux13/1
  uint32Touint8Array28/1(Out1) -> Mux13/2
  Mux13/1 -> [VHAL_DIDSetRESSV2XENNONPSA_raw8]
  Mux14/1 -> [VHAL_DIDSetPKE_raw8]
  uint32Touint8Array30/1(Out1) -> Mux14/2
  uint32Touint8Array29/1(Out1) -> Mux14/1
  uint32Touint8Array31/1(Out1) -> Mux15/1
  uint32Touint8Array32/1(Out1) -> Mux15/2
  Mux15/1 -> [VHAL_DIDSetCDEODT_raw8]
  Mux16/1 -> [VHAL_DIDSetAvgBattTempPSA_raw8]
  Data Type Conversion38/1 -> Mux16/2
  Data Type Conversion37/1 -> Mux16/1
  Data Type Conversion39/1 -> Mux17/1
  Data Type Conversion40/1 -> Mux17/2
  Mux17/1 -> [VHAL_DIDSetAvgBattTempOVC_raw8]
  Mux18/1 -> [VHAL_DIDSetAvgBattTempOFF_raw8]
  Data Type Conversion42/1 -> Mux18/2
  Data Type Conversion41/1 -> Mux18/1
  Mux19/1 -> [VHAL_DIDSetQTYPSATRIPS_raw8]
  uint32Touint8Array34/1(Out1) -> Mux19/2
  uint32Touint8Array33/1(Out1) -> Mux19/1
  uint16Touint8Array21/1(Out1) -> Mux20/8
  uint16Touint8Array20/1(Out1) -> Mux20/7
  uint16Touint8Array19/1(Out1) -> Mux20/6
  uint16Touint8Array18/1(Out1) -> Mux20/5
  uint16Touint8Array17/1(Out1) -> Mux20/4
  uint16Touint8Array16/1(Out1) -> Mux20/3
  uint16Touint8Array15/1(Out1) -> Mux20/2
  uint16Touint8Array14/1(Out1) -> Mux20/1
  Mux20/1 -> [VHAL_DIDSetRESSCNTDODRNGR_raw8]
  Mux21/1 -> [VHAL_DIDSetRESSCNTDODRNGL_raw8]
  uint16Touint8Array22/1(Out1) -> Mux21/1
  uint16Touint8Array23/1(Out1) -> Mux21/2
  uint16Touint8Array24/1(Out1) -> Mux21/3
  uint16Touint8Array25/1(Out1) -> Mux21/4
  uint16Touint8Array26/1(Out1) -> Mux21/5
  uint16Touint8Array27/1(Out1) -> Mux21/6
  uint16Touint8Array28/1(Out1) -> Mux21/7
  uint16Touint8Array29/1(Out1) -> Mux21/8
  Mux22/1 -> [VHAL_DIDSetETMATOE_raw8]
  uint32Touint8Array35/1(Out1) -> Mux22/1
  uint32Touint8Array36/1(Out1) -> Mux22/2
  uint32Touint8Array38/1(Out1) -> Mux23/2
  uint32Touint8Array37/1(Out1) -> Mux23/1
  Mux23/1 -> [VHAL_DIDSetETMBTOE_raw8]
  Mux24/1 -> [VHAL_DIDSetRESSTIMESOCPSARNGR_raw8]
  uint32Touint8Array40/1(Out1) -> Mux24/2
  uint32Touint8Array39/1(Out1) -> Mux24/1
  uint32Touint8Array42/1(Out1) -> Mux24/4
  uint32Touint8Array43/1(Out1) -> Mux24/5
  uint32Touint8Array44/1(Out1) -> Mux24/6
  uint32Touint8Array41/1(Out1) -> Mux24/3
  uint32Touint8Array45/1(Out1) -> Mux24/7
  uint32Touint8Array46/1(Out1) -> Mux24/8
  uint32Touint8Array54/1(Out1) -> Mux25/8
  uint32Touint8Array53/1(Out1) -> Mux25/7
  uint32Touint8Array49/1(Out1) -> Mux25/3
  uint32Touint8Array52/1(Out1) -> Mux25/6
  uint32Touint8Array51/1(Out1) -> Mux25/5
  uint32Touint8Array50/1(Out1) -> Mux25/4
  uint32Touint8Array47/1(Out1) -> Mux25/1
  uint32Touint8Array48/1(Out1) -> Mux25/2
  Mux25/1 -> [VHAL_DIDSetRESSTIMESOCPSARNGL_raw8]
  Mux27/1 -> [VHAL_DIDSetRESSTIMESOCCHGRNGL_raw8]
  uint32Touint8Array64/1(Out1) -> Mux27/2
  uint32Touint8Array63/1(Out1) -> Mux27/1
  uint32Touint8Array66/1(Out1) -> Mux27/4
  uint32Touint8Array67/1(Out1) -> Mux27/5
  uint32Touint8Array68/1(Out1) -> Mux27/6
  uint32Touint8Array65/1(Out1) -> Mux27/3
  uint32Touint8Array69/1(Out1) -> Mux27/7
  uint32Touint8Array70/1(Out1) -> Mux27/8
  uint32Touint8Array62/1(Out1) -> Mux26/8
  uint32Touint8Array61/1(Out1) -> Mux26/7
  uint32Touint8Array57/1(Out1) -> Mux26/3
  uint32Touint8Array60/1(Out1) -> Mux26/6
  uint32Touint8Array59/1(Out1) -> Mux26/5
  uint32Touint8Array58/1(Out1) -> Mux26/4
  uint32Touint8Array55/1(Out1) -> Mux26/1
  uint32Touint8Array56/1(Out1) -> Mux26/2
  Mux26/1 -> [VHAL_DIDSetRESSTIMESOCCHGRNGR_raw8]
  Mux28/1 -> [VHAL_DIDSetRESSTIMESOCOFFRNGR_raw8]
  uint32Touint8Array72/1(Out1) -> Mux28/2
  uint32Touint8Array71/1(Out1) -> Mux28/1
  uint32Touint8Array74/1(Out1) -> Mux28/4
  uint32Touint8Array75/1(Out1) -> Mux28/5
  uint32Touint8Array76/1(Out1) -> Mux28/6
  uint32Touint8Array73/1(Out1) -> Mux28/3
  uint32Touint8Array77/1(Out1) -> Mux28/7
  uint32Touint8Array78/1(Out1) -> Mux28/8
  uint32Touint8Array86/1(Out1) -> Mux29/8
  uint32Touint8Array85/1(Out1) -> Mux29/7
  uint32Touint8Array81/1(Out1) -> Mux29/3
  uint32Touint8Array84/1(Out1) -> Mux29/6
  uint32Touint8Array83/1(Out1) -> Mux29/5
  uint32Touint8Array82/1(Out1) -> Mux29/4
  uint32Touint8Array79/1(Out1) -> Mux29/1
  uint32Touint8Array80/1(Out1) -> Mux29/2
  Mux29/1 -> [VHAL_DIDSetRESSTIMESOCOFFRNGL_raw8]
  [VHAL_DIDSetRUNTM_raw8] -> Bus Creator/19  "VHAL_DIDSetRUNTM_raw8"
  [VHAL_DIDSetVSS_raw8] -> Bus Creator/18  "VHAL_DIDSetVSS_raw8"
  [VHAL_DIDSetMILDIST_raw8] -> Bus Creator/20  "VHAL_DIDSetMILDIST_raw8"
  [VHAL_DIDSetCLRDIST_raw8] -> Bus Creator/22  "VHAL_DIDSetCLRDIST_raw8"
  [VHAL_DIDSetWARMUPS_raw8] -> Bus Creator/21  "VHAL_DIDSetWARMUPS_raw8"
  [VHAL_DIDSetAPPD_raw8] -> Bus Creator/23  "VHAL_DIDSetAPPD_raw8"
  [VHAL_DIDSetAPPE_raw8] -> Bus Creator/24  "VHAL_DIDSetAPPE_raw8"
  [VHAL_DIDSetMILTIME_raw8] -> Bus Creator/25  "VHAL_DIDSetMILTIME_raw8"
  [VHAL_DIDSetCLRTIME_raw8] -> Bus Creator/26  "VHAL_DIDSetCLRTIME_raw8"
  [VHAL_DIDSetBATSOC_raw8] -> Bus Creator/27  "VHAL_DIDSetBATSOC_raw8"
  [VHAL_DIDSetHEVVehSysData_raw8] -> Bus Creator/28  "VHAL_DIDSetHEVVehSysData_raw8"
  [VHAL_DIDSetODOMETER_raw8] -> Bus Creator/29  "VHAL_DIDSetODOMETER_raw8"
  [VHAL_DIDSetBATSOH_raw8] -> Bus Creator/30  "VHAL_DIDSetBATSOH_raw8"
  [VHAL_DIDSetHVBCellVoltMinMax_raw8] -> Bus Creator/31  "VHAL_DIDSetHVBCellVoltMinMax_raw8"
  [VHAL_DIDSetHVESSCHARGE_raw8] -> Bus Creator/32  "VHAL_DIDSetHVESSCHARGE_raw8"
  [VHAL_DIDSetNUMPSATRIPSFLTMEMCLR_raw8] -> Bus Creator/34  "VHAL_DIDSetNUMPSATRIPSFLTMEMCLR_raw8"
  [VHAL_DIDSetHVESSENER_raw8] -> Bus Creator/33  "VHAL_DIDSetHVESSENER_raw8"
  [VHAL_DIDSetHVBattCurr_raw8] -> Bus Creator/35  "VHAL_DIDSetHVBattCurr_raw8"
  [VHAL_DIDSetVIN_raw8] -> Bus Creator/36  "VHAL_DIDSetVIN_raw8"
  [VHAL_DIDSetCALID_raw8] -> Bus Creator/37  "VHAL_DIDSetCALID_raw8"
  [VHAL_DIDSetECUNAME_raw8] -> Bus Creator/38  "VHAL_DIDSetECUNAME_raw8"
  [VHAL_DIDSetProtocolId_raw8] -> Bus Creator/39  "VHAL_DIDSetProtocolId_raw8"
  [VHAL_DIDSetPSA_raw8] -> Bus Creator/40  "VHAL_DIDSetPSA_raw8"
  [VHAL_DIDSetTNBCPSA_raw8] -> Bus Creator/41  "VHAL_DIDSetTNBCPSA_raw8"
  [VHAL_DIDSetTNECPSA_raw8] -> Bus Creator/42  "VHAL_DIDSetTNECPSA_raw8"
  [VHAL_DIDSetTEBPSA_raw8] -> Bus Creator/43  "VHAL_DIDSetTEBPSA_raw8"
  [VHAL_DIDSetTGEOVC_raw8] -> Bus Creator/44  "VHAL_DIDSetTGEOVC_raw8"
  [VHAL_DIDSetGECHGOVCDC_raw8] -> Bus Creator/45  "VHAL_DIDSetGECHGOVCDC_raw8"
  [VHAL_DIDSetGECHGOVCAC_raw8] -> Bus Creator/46  "VHAL_DIDSetGECHGOVCAC_raw8"
  [VHAL_DIDSetRESSV2XENNONPSA_raw8] -> Bus Creator/47  "VHAL_DIDSetRESSV2XENNONPSA_raw8"
  [VHAL_DIDSetPKE_raw8] -> Bus Creator/48  "VHAL_DIDSetPKE_raw8"
  [VHAL_DIDSetCDEODT_raw8] -> Bus Creator/49  "VHAL_DIDSetCDEODT_raw8"
  [VHAL_DIDSetAvgBattTempPSA_raw8] -> Bus Creator/50  "VHAL_DIDSetAvgBattTempPSA_raw8"
  [VHAL_DIDSetAvgBattTempOVC_raw8] -> Bus Creator/51  "VHAL_DIDSetAvgBattTempOVC_raw8"
  [VHAL_DIDSetAvgBattTempOFF_raw8] -> Bus Creator/52  "VHAL_DIDSetAvgBattTempOFF_raw8"
  [VHAL_DIDSetQTYPSATRIPS_raw8] -> Bus Creator/53  "VHAL_DIDSetQTYPSATRIPS_raw8"
  [VHAL_DIDSetRESSCNTDODRNGR_raw8] -> Bus Creator/54  "VHAL_DIDSetRESSCNTDODRNGR_raw8"
  [VHAL_DIDSetRESSCNTDODRNGL_raw8] -> Bus Creator/55  "VHAL_DIDSetRESSCNTDODRNGL_raw8"
  [VHAL_DIDSetETMATOE_raw8] -> Bus Creator/56  "VHAL_DIDSetETMATOE_raw8"
  [VHAL_DIDSetETMBTOE_raw8] -> Bus Creator/57  "VHAL_DIDSetETMBTOE_raw8"
  [VHAL_DIDSetRESSTIMESOCPSARNGR_raw8] -> Bus Creator/58  "VHAL_DIDSetRESSTIMESOCPSARNGR_raw8"
  [VHAL_DIDSetRESSTIMESOCPSARNGL_raw8] -> Bus Creator/59  "VHAL_DIDSetRESSTIMESOCPSARNGL_raw8"
  [VHAL_DIDSetRESSTIMESOCCHGRNGR_raw8] -> Bus Creator/60  "VHAL_DIDSetRESSTIMESOCCHGRNGR_raw8"
  [VHAL_DIDSetRESSTIMESOCCHGRNGL_raw8] -> Bus Creator/61  "VHAL_DIDSetRESSTIMESOCCHGRNGL_raw8"
  [VHAL_DIDSetRESSTIMESOCOFFRNGL_raw8] -> Bus Creator/63  "VHAL_DIDSetRESSTIMESOCOFFRNGL_raw8"
  [VHAL_DIDSetRESSTIMESOCOFFRNGR_raw8] -> Bus Creator/62  "VHAL_DIDSetRESSTIMESOCOFFRNGR_raw8"
  Data Type Conversion43/1 -> Terminator_1/1
  Data Type Conversion44/1 -> Terminator_2/1
  Data Type Conversion45/1 -> Terminator_3/1
  uint16Touint8Array13/1(Out1) -> Terminator_4/1
  uint32Touint8Array13/1(Out1) -> Terminator_5/1
  uint32Touint8Array14/1(Out1) -> Terminator_6/1
  convert_in/1 -> uint32Touint8Array4/1(In1)
  [VOUTP_ODOMETER_km] -> convert_in/1
  [VOUTP_HVBNAH_Ahr] -> convert_in1/1
  convert_in1/1 -> uint32Touint8Array13/1(In1)
  convert_in2/1 -> uint32Touint8Array14/1(In1)
  [VOUTP_HVBNE_kWh] -> convert_in2/1
  [VOUTP_TEBPSAR_kWh] -> convert_in5/1
  [VOUTP_TNECPSAR_kWh] -> convert_in19/1
  [VOUTP_TNECPSAL_kWh] -> convert_in18/1
  [VOUTP_TEBPSAL_kWh] -> convert_in17/1
  [VOUTP_TGEOVCR_kWh] -> convert_in6/1
  [VOUTP_TGEOVCL_kWh] -> convert_in7/1
  [VOUTP_GECHGOVCDCR_kWh] -> convert_in8/1
  [VOUTP_GECHGOVCDCL_kWh] -> convert_in9/1
  [VOUTP_GECHGOVCACL_kWh] -> convert_in21/1
  [VOUTP_GECHGOVCACR_kWh] -> convert_in20/1
  [VOUTP_RESSV2XENNONPSAR_kWh] -> convert_in10/1
  [VOUTP_RESSV2XENNONPSAL_kWh] -> convert_in11/1
  [VOUTP_CDEODTR_km] -> convert_in12/1
  [VOUTP_CDEODTL_km] -> convert_in13/1
  [VOUTP_AvgBattTempPSAR_C] -> convert_in14/1
  convert_in14/1 -> Data Type Conversion37/1
  convert_in15/1 -> Data Type Conversion38/1
  [VOUTP_AvgBattTempPSAL_C] -> convert_in15/1
  [VOUTP_AvgBattTempOVCL_C] -> convert_in22/1
  convert_in22/1 -> Data Type Conversion40/1
  convert_in16/1 -> Data Type Conversion39/1
  [VOUTP_AvgBattTempOVCR_C] -> convert_in16/1
  [VOUTP_AvgBattTempOFFR_C] -> convert_in23/1
  convert_in23/1 -> Data Type Conversion41/1
  convert_in24/1 -> Data Type Conversion42/1
  [VOUTP_AvgBattTempOFFL_C] -> convert_in24/1
  [VOUTP_HVBATT_A] -> convert_in25/1
  convert_in25/1 -> uint16Touint8Array7/1(In1)
  convert_in26/1 -> uint16Touint8Array6/1(In1)
  [VOUTP_HEVBATT_V] -> convert_in26/1
  convert_in27/1 -> Data Type Conversion28/1
  [VOUTP_BATSOC_pct] -> convert_in27/1
  [VOUTP_APPE_pct] -> convert_in28/1
  convert_in28/1 -> Data Type Conversion29/1
  convert_in29/1 -> Data Type Conversion27/1
  [VOUTP_APPD_pct] -> convert_in29/1
  [VOUTP_BATSOH_pct] -> convert_in30/1
  convert_in30/1 -> Data Type Conversion32/1
  [VOUTP_HVBCellVoltMin_V] -> convert_in31/1
  convert_in31/1 -> uint16Touint8Array8/1(In1)
  convert_in32/1 -> uint16Touint8Array9/1(In1)
  [VOUTP_HVBCellVoltMax_V] -> convert_in32/1
  convert_in33/1 -> uint16Touint8Array10/1(In1)
  convert_in34/1 -> uint16Touint8Array11/1(In1)
  [VOUTP_HVESSCHARGEACT_kW] -> convert_in34/1
  [VOUTP_HVESSCHARGELIM_kW] -> convert_in33/1
  [VOUTP_HVBattCurr_Ahps] -> convert_in36/1
  convert_in36/1 -> uint32Touint8Array6/1(In1)
  [VOUTP_HVESSENER_Whps] -> convert_in35/1
  convert_in35/1 -> uint32Touint8Array5/1(In1)
  [VOUTP_TNBCPSAL_Ahr] -> convert_in4/1
  [VOUTP_TNBCPSAR_Ahr] -> convert_in3/1
  convert_out101/1 -> UnitConverter449/1
  SignalPack345/1 -> UnitConverter439/1
  [DKCFDCDKCCoordinateYSta] -> convert_out101/1
  SignalPack344/1 -> UnitConverter438/1
  UnitConverter274/1 -> Mux48/11
  UnitConverter270/1 -> Mux48/9
  UnitConverter258/1 -> Mux48/3
  convert_out98/1 -> UnitConverter440/1
  SignalPack350/1 -> UnitConverter447/1
  UnitConverter413/1 -> SignalPack323/1
  Mux55/1 -> [VHAL_DIDSetDoorNFCanchorStatus_raw8]
  convert_out94/1 -> UnitConverter413/1
  [DKCDooranchorDetectedNFCcard] -> convert_out94/1
  SignalPack183/1 -> UnitConverter242/1
  UnitConverter240/1 -> BitwiseAND/2
  convert_out57/1 -> UnitConverter239/1
  [CurrentKeyfobposition] -> convert_out57/1
  convert_out56/1 -> UnitConverter237/1
  SignalPack199/1 -> UnitConverter274/1
  SignalPack189/1 -> UnitConverter254/1
  UnitConverter246/1 -> Mux38/2
  Mux61/1 -> [VHAL_DIDSetUIDStatus_raw8]
  UnitConverter264/1 -> Mux48/6
  UnitConverter269/1 -> SignalPack197/1
  [DKCDKCUWB4FPPSta] -> convert_out72/1
  SignalPack185/1 -> UnitConverter246/1
  UnitConverter265/1 -> SignalPack195/1
  convert_out77/1 -> UnitConverter275/1
  SignalPack193/1 -> UnitConverter262/1
  UnitConverter271/1 -> SignalPack198/1
  UnitConverter267/1 -> SignalPack196/1
  UnitConverter238/1 -> BitwiseAND/1
  UnitConverter244/1 -> Mux38/1
  convert_out74/1 -> UnitConverter269/1
  UnitConverter256/1 -> BitwiseAND1/4
  convert_out70/1 -> UnitConverter263/1
  [DKCDKCUWB3FPPSta] -> convert_out70/1
  convert_out75/1 -> UnitConverter271/1
  SignalPack190/1 -> UnitConverter256/1
  Mux38/1 -> [VHAL_DIDSetBLEStatus_raw8]
  SignalPack186/1 -> UnitConverter248/1
  [DKCUWB3InvalidSta] -> convert_out65/1
  UnitConverter247/1 -> SignalPack186/1
  convert_out58/1 -> UnitConverter241/1
  UnitConverter243/1 -> SignalPack184/1
  [DKCBLERSSI] -> convert_out61/1
  UnitConverter257/1 -> SignalPack191/1
  convert_out78/1 -> UnitConverter277/1
  SignalPack200/1 -> UnitConverter276/1
  UnitConverter261/1 -> SignalPack193/1
  UnitConverter255/1 -> SignalPack190/1
  convert_out76/1 -> UnitConverter273/1
  UnitConverter439/1 -> Mux58/2
  [DKCUIDcurrentvoltage] -> convert_out97/1
  SignalPack353/1 -> UnitConverter451/1
  SignalPack302/1 -> UnitConverter390/1
  UnitConverter389/1 -> SignalPack302/1
  convert_out72/1 -> UnitConverter265/1
  SignalPack182/1 -> UnitConverter240/1
  convert_out64/1 -> UnitConverter251/1
  SignalPack184/1 -> UnitConverter244/1
  UnitConverter250/1 -> BitwiseAND1/1
  [DKCFDCDKCCoordinateXSta] -> convert_out100/1
  SignalPack187/1 -> UnitConverter250/1
  Mux59/1 -> Mux61/4
  Mux60/1 -> Mux61/5
  SignalPack348/1 -> UnitConverter444/1
  SignalPack349/1 -> UnitConverter445/1
  UnitConverter445/1 -> Mux60/2
  UnitConverter253/1 -> SignalPack189/1
  UnitConverter449/1 -> SignalPack352/1, SignalPack353/1
  SignalPack197/1 -> UnitConverter270/1
  UnitConverter446/1 -> SignalPack350/1, SignalPack351/1
  UnitConverter442/1 -> Mux59/2
  UnitConverter278/1 -> Mux48/13
  convert_out90/1 -> UnitConverter389/1
  [DKCLIDAanchorDetectedNFCcard] -> convert_out90/1
  Mux65/1 -> [VHAL_DIDSetFDDKCCoordinateXY_raw8]
  UnitConverter237/1 -> SignalPack181/1
  UnitConverter263/1 -> SignalPack194/1
  UnitConverter441/1 -> Mux59/1
  [DKCUIDMinvoltage] -> convert_out99/1
  [DKCKW45moduleresetevent] -> convert_out58/1
  UnitConverter260/1 -> Mux48/4
  [DKCDKCUWB1DistanceSta] -> convert_out74/1
  Mux58/1 -> Mux61/3
  UnitConverter254/1 -> BitwiseAND1/3
  convert_out99/1 -> UnitConverter443/1
  convert_out68/1 -> UnitConverter259/1
  Mux36/1 -> [VHAL_DIDSetReadKeyIndexDataIdentifier_raw8]
  UnitConverter390/1 -> Mux51/3
  UnitConverter262/1 -> Mux48/5
  [DKCDKCUWB2DistanceSta] -> convert_out75/1
  convert_out69/1 -> UnitConverter261/1
  [DKCDKCUWB2FPPSta] -> convert_out69/1
  SignalPack323/1 -> UnitConverter414/1
  Mux51/1 -> [VHAL_DIDSetLIDAanchorStatus_raw8]
  [DKCBLElossCounter] -> convert_out59/1
  BitwiseAND/1 -> Mux37/1
  SignalPack201/1 -> UnitConverter278/1
  UnitConverter266/1 -> Mux48/7
  [DKCUWB2InvalidSta] -> convert_out64/1
  [CurrentCarKeytype] -> convert_out56/1
  SignalPack346/1 -> UnitConverter441/1
  UnitConverter444/1 -> Mux60/1
  convert_out59/1 -> UnitConverter243/1
  SignalPack198/1 -> UnitConverter272/1
  SignalPack351/1 -> UnitConverter448/1
  UnitConverter249/1 -> SignalPack187/1
  Mux37/1 -> [VHAL_DIDSetDKCStatus_raw8]
  UnitConverter443/1 -> SignalPack348/1, SignalPack349/1
  SignalPack352/1 -> UnitConverter450/1
  [DKCDKCUWB1FPPSta] -> convert_out68/1
  UnitConverter259/1 -> SignalPack192/1
  SignalPack188/1 -> UnitConverter252/1
  UnitConverter252/1 -> BitwiseAND1/2
  UnitConverter251/1 -> SignalPack188/1
  convert_out66/1 -> UnitConverter255/1
  [DKCUWB4InvalidSta] -> convert_out66/1
  convert_out62/1 -> UnitConverter247/1
  [DKCDKCUWBOnOffSta] -> convert_out62/1
  convert_out73/1 -> UnitConverter267/1
  convert_out63/1 -> UnitConverter249/1
  UnitConverter248/1 -> Mux48/1
  UnitConverter437/1 -> SignalPack344/1, SignalPack345/1
  UnitConverter242/1 -> Mux37/2
  convert_out65/1 -> UnitConverter253/1
  [DKCDKCUWB4DistanceSta] -> convert_out77/1
  UnitConverter276/1 -> Mux48/12
  UnitConverter275/1 -> SignalPack200/1
  BitwiseAND1/1 -> Mux48/2
  UnitConverter438/1 -> Mux58/1
  SignalPack347/1 -> UnitConverter442/1
  convert_out100/1 -> UnitConverter446/1
  SignalPack194/1 -> UnitConverter264/1
  [BOUTP_outputs] -> bus_selector/1
  UnitConverter273/1 -> SignalPack199/1
  UnitConverter245/1 -> SignalPack185/1
  convert_out61/1 -> UnitConverter245/1
  SignalPack195/1 -> UnitConverter266/1
  UnitConverter268/1 -> Mux48/8
  SignalPack196/1 -> UnitConverter268/1
  convert_out97/1 -> UnitConverter437/1
  [DKCDKCUWB3DistanceSta] -> convert_out76/1
  UnitConverter414/1 -> Mux55/3
  [DKCUWB1InvalidSta] -> convert_out63/1
  [DKCDKCUWB5InvalidSta] -> convert_out67/1
  SignalPack192/1 -> UnitConverter260/1
  [DKCDKCUWB5DistanceSta] -> convert_out78/1
  Mux48/1 -> [VHAL_DIDSetUWBanchorStatus_raw8]
  UnitConverter239/1 -> SignalPack182/1
  UnitConverter272/1 -> Mux48/10
  convert_out67/1 -> UnitConverter257/1
  UnitConverter241/1 -> SignalPack183/1
  SignalPack191/1 -> UnitConverter258/1
  [DKCDKCUWB5FPPSta] -> convert_out73/1
  UnitConverter277/1 -> SignalPack201/1
  UnitConverter440/1 -> SignalPack346/1, SignalPack347/1
  SignalPack181/1 -> UnitConverter238/1
  [DKCUIDMaxvoltage] -> convert_out98/1
  BOUTP_outputs/1 -> [BOUTP_outputs]
  [BOUTP_outputs] -> Bus Selector/1
  [VHAL_DIDSetReadKeyIndexDataIdentifier_raw8] -> Bus Creator/64  "VHAL_DIDSetReadKeyIndexDataIdentifier_raw8"
  [VHAL_DIDSetDKCStatus_raw8] -> Bus Creator/65  "VHAL_DIDSetDKCSta_raw8"
  [VHAL_DIDSetBLEStatus_raw8] -> Bus Creator/66  "VHAL_DIDSetDKCBLESta_raw8"
  [VHAL_DIDSetUWBanchorStatus_raw8] -> Bus Creator/67  "VHAL_DIDSetUWBAnchorSta_raw8"
  [VHAL_DIDSetLIDAanchorStatus_raw8] -> Bus Creator/68  "VHAL_DIDSetLIDAAnchorSta_raw8"
  [VHAL_DIDSetDoorNFCanchorStatus_raw8] -> Bus Creator/69  "VHAL_DIDSetDoorNFCAnchorSta_raw8"
  [VHAL_DIDSetUIDStatus_raw8] -> Bus Creator/70  "VHAL_DIDSetUIDSta_raw8"
  [VHAL_DIDSetFDDKCCoordinateXY_raw8] -> Bus Creator/71  "VHAL_DIDSetFDDKCCoordXY_raw8"
  bus_selector/1 -> [CurrentCarKeytype]  "<VOUTP_KeyModeSta_enum>"
  bus_selector/2 -> [CurrentKeyfobposition]  "<VOUTP_UWBDetArea_enum>"
  bus_selector/3 -> [DKCBLERSSI]  "<VOUTP_BLERSSI_enum>"
  bus_selector/4 -> [DKCDKCUWBOnOffSta]  "<VOUTP_UWBOnOff_flg>"
  bus_selector/5 -> [DKCUWB1InvalidSta]  "<VOUTP_UWB1Invalid_flg>"
  bus_selector/6 -> [DKCUWB2InvalidSta]  "<VOUTP_UWB2Invalid_flg>"
  bus_selector/7 -> [DKCUWB3InvalidSta]  "<VOUTP_UWB3Invalid_flg>"
  bus_selector/8 -> [DKCUWB4InvalidSta]  "<VOUTP_UWB4Invalid_flg>"
  bus_selector/9 -> [DKCDKCUWB5InvalidSta]  "<VOUTP_UWB0Invalid_flg>"
  bus_selector/10 -> [DKCDKCUWB1FPPSta]  "<VOUTP_UWB1FPP_enum>"
  bus_selector/11 -> [DKCDKCUWB2FPPSta]  "<VOUTP_UWB2FPP_enum>"
  bus_selector/12 -> [DKCDKCUWB3FPPSta]  "<VOUTP_UWB3FPP_enum>"
  bus_selector/13 -> [DKCDKCUWB4FPPSta]  "<VOUTP_UWB4FPP_enum>"
  bus_selector/14 -> [DKCDKCUWB5FPPSta]  "<VOUTP_UWB0FPP_enum>"
  bus_selector/15 -> [DKCDKCUWB1DistanceSta]  "<VOUTP_UWB1Distance_enum>"
  bus_selector/16 -> [DKCDKCUWB2DistanceSta]  "<VOUTP_UWB2Distance_enum>"
  bus_selector/17 -> [DKCDKCUWB3DistanceSta]  "<VOUTP_UWB3Distance_enum>"
  bus_selector/18 -> [DKCDKCUWB4DistanceSta]  "<VOUTP_UWB4Distance_enum>"
  bus_selector/19 -> [DKCDKCUWB5DistanceSta]  "<VOUTP_UWB0Distance_enum>"
  bus_selector/20 -> [DKCUIDcurrentvoltage]  "<VOUTP_UIDBatVolt_enum>"
  bus_selector/21 -> [DKCFDCDKCCoordinateXSta]  "<VOUTP_CoordinateX_enum>"
  bus_selector/22 -> [DKCFDCDKCCoordinateYSta]  "<VOUTP_CoordinateY_enum>"
  [DKCUWB1anchorHardwareVersion] -> Mux48/14
  [DKCUWB1anchorSoftwareVersion] -> Mux48/15
  [DKCUWB2anchorHardwareVersion] -> Mux48/16
  [DKCUWB2anchorSoftwareVersion] -> Mux48/17
  [DKCUWB3anchorHardwareVersion] -> Mux48/18
  [DKCUWB3anchorSoftwareVersion] -> Mux48/19
  [DKCUWB4anchorHardwareVersion] -> Mux48/20
  [DKCUWB4anchorSoftwareVersion] -> Mux48/21
  [DKCLIDAanchorHardwareVersion] -> Mux51/1
  [DKCLIDAanchorSoftwareVersion] -> Mux51/2
  [DKCDooranchorHardwareVersion] -> Mux55/1
  [DKCDooranchorSoftwareVersion] -> Mux55/2
  [DKCUIDHardwareVersion] -> Mux61/1
  [DKCUIDSoftwareVersion] -> Mux61/2
  UnitConverter448/1 -> BitwiseAND2/1
  UnitConverter450/1 -> BitwiseAND2/2
  BitwiseAND2/1 -> Mux65/2
  UnitConverter447/1 -> Mux65/1
  UnitConverter451/1 -> Mux65/3
  Constant3/1 -> Data Type Conversion46/1
  Constant4/1 -> Data Type Conversion/1
  Constant5/1 -> Data Type Conversion47/1
  Constant6/1 -> Data Type Conversion48/1
  Constant7/1 -> Data Type Conversion49/1
  Constant8/1 -> Data Type Conversion50/1
  Constant9/1 -> Data Type Conversion51/1
  Constant10/1 -> Data Type Conversion52/1
  Constant11/1 -> Data Type Conversion53/1
  Constant12/1 -> Data Type Conversion54/1
  Constant13/1 -> Data Type Conversion55/1
  Constant14/1 -> Data Type Conversion56/1
  Constant15/1 -> Data Type Conversion57/1
  Constant16/1 -> Data Type Conversion58/1
  Data Type Conversion/1 -> [DKCUWB1anchorSoftwareVersion]
  Data Type Conversion46/1 -> [DKCUWB1anchorHardwareVersion]
  Data Type Conversion47/1 -> [DKCUWB2anchorHardwareVersion]
  Data Type Conversion48/1 -> [DKCUWB2anchorSoftwareVersion]
  Data Type Conversion49/1 -> [DKCUWB3anchorHardwareVersion]
  Data Type Conversion52/1 -> [DKCUWB4anchorSoftwareVersion]
  Data Type Conversion51/1 -> [DKCUWB4anchorHardwareVersion]
  Data Type Conversion50/1 -> [DKCUWB3anchorSoftwareVersion]
  Data Type Conversion53/1 -> [DKCLIDAanchorHardwareVersion]
  Data Type Conversion54/1 -> [DKCLIDAanchorSoftwareVersion]
  Data Type Conversion55/1 -> [DKCDooranchorHardwareVersion]
  Data Type Conversion56/1 -> [DKCDooranchorSoftwareVersion]
  Data Type Conversion57/1 -> [DKCUIDHardwareVersion]
  Data Type Conversion58/1 -> [DKCUIDSoftwareVersion]
